simulink model "Filter_Sim_10th_Order"  (R2017a)
settings: Solver=VariableStepAuto  StartTime=0.0  StopTime=t_stop  RelTol=1e-3
values from neighbouring files (symbols this model uses):
  ts = 1/fs    (= 8.85770975057e-08)    [Filter_Sim.m]
libraries: Bitstream_Library x2
settings Model: Creator=jpoverelli  LastModifiedBy=jpoverelli

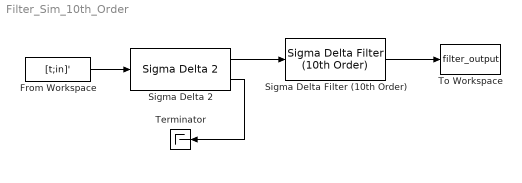
== system Filter_Sim_10th_Order ==
  From Workspace : FromWorkspace  VariableName=[t;in]'  SampleTime=ts
  Sigma Delta 2 : Bitstream_Library/Sigma Delta 2
  Sigma Delta Filter (10th Order) : Bitstream_Library/Sigma Delta Filter (10th Order)
  Terminator : Terminator
  To Workspace : ToWorkspace  VariableName=filter_output  SampleTime=-1
  wires:
  From Workspace/1 -> Sigma Delta 2/1
  Sigma Delta 2/2 -> Terminator/1
  Sigma Delta 2/1 -> Sigma Delta Filter (10th Order)/1
  Sigma Delta Filter (10th Order)/1 -> To Workspace/1
